simulink model "system_20220515_1_sm_master"  (R2020b)
settings: Solver=ode4  StartTime=0.0  StopTime=inf  FixedStep=0.001  RelTol=1e-3  EnableMultiTasking=on
PreLoadFcn:
  | simulation_vars
PostLoadFcn:
  | simulation_vars
InitFcn:
  | simulation_vars
StartFcn:
  | simulation_vars
undefined symbols (not defined in the file or in its folder): ang_variance, bus_va_seed, bus_vm_seed, en_spoofing_attack, event_time_end, event_time_start, line_iang0_seed, line_iang1_seed, line_imag0_seed, line_imag1_seed, mag_variance, spoof_lower_limit, spoof_upper_limit, Ts, xf_iang0_seed, xf_iang1_seed, xf_imag0_seed, xf_imag1_seed
libraries: rtlab x209, simulink x21, opal_lib x3, rtlab_phasor x1, rtio_spectracom x1
(part 4 of 4)

== system system_20220515_1_sm_master/sm_master/PMU207_signals/Spoofing attack ==
  note: Modify demux and mux to fit input size.
      | Only modifies the angle measurements.
  Input : Inport
  Add : Sum
  Constant : Constant  Value=en_spoofing_attack.pmu_207
  Demux : Demux
  Demux1 : Demux  Outputs=2
  Multiply : Product
  Mux : Mux
  Mux1 : Mux  Inputs=2
  Ramp : simulink/Sources/Ramp  slope=1*pi()/180  start=spoof_st.pmu_207  InitialOutput=0
  Saturation : Saturate  UpperLimit=spoof_upper_limit  LowerLimit=spoof_lower_limit
  Output : Outport  VectorParamsAs1DForOutWhenUnconnected=off
  wires:
  Multiply/1 -> Add/1
  Saturation/1 -> Multiply/1
  Constant/1 -> Multiply/2
  Ramp/1 -> Saturation/1
  Input/1 -> Demux/1
  Mux/1 -> Output/1
  Demux/1 -> Mux/1
  Demux/3 -> Mux/3
  Demux/4 -> Mux1/2
  Demux/2 -> Mux1/1
  Mux1/1 -> Add/2
  Add/1 -> Demux1/1
  Demux1/1 -> Mux/2
  Demux1/2 -> Mux/4

== system system_20220515_1_sm_master/sm_master/PMU210_signals/Spoofing attack ==
  note: Modify demux and mux to fit input size.
      | Only modifies the angle measurements.
  Input : Inport
  Add : Sum
  Constant : Constant  Value=en_spoofing_attack.pmu_210
  Demux : Demux  Outputs=12
  Demux1 : Demux  Outputs=6
  Multiply : Product
  Mux : Mux  Inputs=12
  Mux1 : Mux  Inputs=6
  Ramp : simulink/Sources/Ramp  slope=1*pi()/180  start=spoof_st.pmu_210  InitialOutput=0
  Saturation : Saturate  UpperLimit=spoof_upper_limit  LowerLimit=spoof_lower_limit
  Output : Outport  VectorParamsAs1DForOutWhenUnconnected=off
  wires:
  Multiply/1 -> Add/1
  Saturation/1 -> Multiply/1
  Constant/1 -> Multiply/2
  Ramp/1 -> Saturation/1
  Input/1 -> Demux/1
  Mux/1 -> Output/1
  Demux/1 -> Mux/1
  Demux/3 -> Mux/3
  Demux/5 -> Mux/5
  Demux/7 -> Mux/7
  Demux/9 -> Mux/9
  Demux/10 -> Mux1/5
  Demux/8 -> Mux1/4
  Demux/6 -> Mux1/3
  Demux/4 -> Mux1/2
  Demux/2 -> Mux1/1
  Mux1/1 -> Add/2
  Add/1 -> Demux1/1
  Demux1/1 -> Mux/2
  Demux1/2 -> Mux/4
  Demux1/3 -> Mux/6
  Demux1/4 -> Mux/8
  Demux1/5 -> Mux/10
  Demux/11 -> Mux/11
  Demux/12 -> Mux1/6
  Demux1/6 -> Mux/12

== system system_20220515_1_sm_master/sm_master/PMU216_signals/Spoofing attack ==
  note: Modify demux and mux to fit input size.
      | Only modifies the angle measurements.
  Input : Inport
  Add : Sum
  Constant : Constant  Value=en_spoofing_attack.pmu_216
  Demux : Demux  Outputs=10
  Demux1 : Demux  Outputs=5
  Multiply : Product
  Mux : Mux  Inputs=10
  Mux1 : Mux  Inputs=5
  Ramp : simulink/Sources/Ramp  slope=1*pi()/180  start=spoof_st.pmu_216  InitialOutput=0
  Saturation : Saturate  UpperLimit=spoof_upper_limit  LowerLimit=spoof_lower_limit
  Output : Outport  VectorParamsAs1DForOutWhenUnconnected=off
  wires:
  Multiply/1 -> Add/1
  Saturation/1 -> Multiply/1
  Constant/1 -> Multiply/2
  Ramp/1 -> Saturation/1
  Input/1 -> Demux/1
  Mux/1 -> Output/1
  Demux/1 -> Mux/1
  Demux/3 -> Mux/3
  Demux/5 -> Mux/5
  Demux/7 -> Mux/7
  Demux/9 -> Mux/9
  Demux/10 -> Mux1/5
  Demux/8 -> Mux1/4
  Demux/6 -> Mux1/3
  Demux/4 -> Mux1/2
  Demux/2 -> Mux1/1
  Mux1/1 -> Add/2
  Add/1 -> Demux1/1
  Demux1/1 -> Mux/2
  Demux1/2 -> Mux/4
  Demux1/3 -> Mux/6
  Demux1/4 -> Mux/8
  Demux1/5 -> Mux/10

== system system_20220515_1_sm_master/sm_master/PMU221_signals/Spoofing attack ==
  note: Modify demux and mux to fit input size.
      | Only modifies the angle measurements.
  Input : Inport
  Add : Sum
  Constant : Constant  Value=en_spoofing_attack.pmu_221
  Demux : Demux  Outputs=12
  Demux1 : Demux  Outputs=6
  Multiply : Product
  Mux : Mux  Inputs=12
  Mux1 : Mux  Inputs=6
  Ramp : simulink/Sources/Ramp  slope=1*pi()/180  start=spoof_st.pmu_221  InitialOutput=0
  Saturation : Saturate  UpperLimit=spoof_upper_limit  LowerLimit=spoof_lower_limit
  Output : Outport  VectorParamsAs1DForOutWhenUnconnected=off
  wires:
  Multiply/1 -> Add/1
  Saturation/1 -> Multiply/1
  Constant/1 -> Multiply/2
  Ramp/1 -> Saturation/1
  Input/1 -> Demux/1
  Mux/1 -> Output/1
  Demux/1 -> Mux/1
  Demux/3 -> Mux/3
  Demux/5 -> Mux/5
  Demux/7 -> Mux/7
  Demux/9 -> Mux/9
  Demux/10 -> Mux1/5
  Demux/8 -> Mux1/4
  Demux/6 -> Mux1/3
  Demux/4 -> Mux1/2
  Demux/2 -> Mux1/1
  Mux1/1 -> Add/2
  Add/1 -> Demux1/1
  Demux1/1 -> Mux/2
  Demux1/2 -> Mux/4
  Demux1/3 -> Mux/6
  Demux1/4 -> Mux/8
  Demux1/5 -> Mux/10
  Demux/11 -> Mux/11
  Demux/12 -> Mux1/6
  Demux1/6 -> Mux/12

== system system_20220515_1_sm_master/sm_master/PMU223_signals/Spoofing attack ==
  note: Modify demux and mux to fit input size.
      | Only modifies the angle measurements.
  Input : Inport
  Add : Sum
  Constant : Constant  Value=en_spoofing_attack.pmu_223
  Demux : Demux  Outputs=12
  Demux1 : Demux  Outputs=6
  Multiply : Product
  Mux : Mux  Inputs=12
  Mux1 : Mux  Inputs=6
  Ramp : simulink/Sources/Ramp  slope=1*pi()/180  start=spoof_st.pmu_223  InitialOutput=0
  Saturation : Saturate  UpperLimit=spoof_upper_limit  LowerLimit=spoof_lower_limit
  Output : Outport  VectorParamsAs1DForOutWhenUnconnected=off
  wires:
  Multiply/1 -> Add/1
  Saturation/1 -> Multiply/1
  Constant/1 -> Multiply/2
  Ramp/1 -> Saturation/1
  Input/1 -> Demux/1
  Mux/1 -> Output/1
  Demux/1 -> Mux/1
  Demux/3 -> Mux/3
  Demux/5 -> Mux/5
  Demux/7 -> Mux/7
  Demux/9 -> Mux/9
  Demux/10 -> Mux1/5
  Demux/8 -> Mux1/4
  Demux/6 -> Mux1/3
  Demux/4 -> Mux1/2
  Demux/2 -> Mux1/1
  Mux1/1 -> Add/2
  Add/1 -> Demux1/1
  Demux1/1 -> Mux/2
  Demux1/2 -> Mux/4
  Demux1/3 -> Mux/6
  Demux1/4 -> Mux/8
  Demux1/5 -> Mux/10
  Demux/11 -> Mux/11
  Demux/12 -> Mux1/6
  Demux1/6 -> Mux/12

== system system_20220515_1_sm_master/sm_master/PMU302_signals/Spoofing attack ==
  note: Modify demux and mux to fit input size.
      | Only modifies the angle measurements.
  Input : Inport
  Add : Sum
  Constant : Constant  Value=en_spoofing_attack.pmu_302
  Demux : Demux  Outputs=8
  Demux1 : Demux
  Multiply : Product
  Mux : Mux  Inputs=8
  Mux1 : Mux
  Ramp : simulink/Sources/Ramp  slope=1*pi()/180  start=spoof_st.pmu_302  InitialOutput=0
  Saturation : Saturate  UpperLimit=spoof_upper_limit  LowerLimit=spoof_lower_limit
  Output : Outport  VectorParamsAs1DForOutWhenUnconnected=off
  wires:
  Multiply/1 -> Add/1
  Saturation/1 -> Multiply/1
  Constant/1 -> Multiply/2
  Ramp/1 -> Saturation/1
  Input/1 -> Demux/1
  Mux/1 -> Output/1
  Demux/1 -> Mux/1
  Demux/3 -> Mux/3
  Demux/5 -> Mux/5
  Demux/7 -> Mux/7
  Demux/8 -> Mux1/4
  Demux/6 -> Mux1/3
  Demux/4 -> Mux1/2
  Demux/2 -> Mux1/1
  Mux1/1 -> Add/2
  Add/1 -> Demux1/1
  Demux1/1 -> Mux/2
  Demux1/2 -> Mux/4
  Demux1/3 -> Mux/6
  Demux1/4 -> Mux/8

== system system_20220515_1_sm_master/sm_master/PMU303_signals/Spoofing attack ==
  note: Modify demux and mux to fit input size.
      | Only modifies the angle measurements.
  Input : Inport
  Add : Sum
  Constant : Constant  Value=en_spoofing_attack.pmu_303
  Demux : Demux  Outputs=8
  Demux1 : Demux
  Multiply : Product
  Mux : Mux  Inputs=8
  Mux1 : Mux
  Ramp : simulink/Sources/Ramp  slope=1*pi()/180  start=spoof_st.pmu_303  InitialOutput=0
  Saturation : Saturate  UpperLimit=spoof_upper_limit  LowerLimit=spoof_lower_limit
  Output : Outport  VectorParamsAs1DForOutWhenUnconnected=off
  wires:
  Multiply/1 -> Add/1
  Saturation/1 -> Multiply/1
  Constant/1 -> Multiply/2
  Ramp/1 -> Saturation/1
  Input/1 -> Demux/1
  Mux/1 -> Output/1
  Demux/1 -> Mux/1
  Demux/3 -> Mux/3
  Demux/5 -> Mux/5
  Demux/7 -> Mux/7
  Demux/8 -> Mux1/4
  Demux/6 -> Mux1/3
  Demux/4 -> Mux1/2
  Demux/2 -> Mux1/1
  Mux1/1 -> Add/2
  Add/1 -> Demux1/1
  Demux1/1 -> Mux/2
  Demux1/2 -> Mux/4
  Demux1/3 -> Mux/6
  Demux1/4 -> Mux/8

== system system_20220515_1_sm_master/sm_master/PMU307_signals/Spoofing attack ==
  note: Modify demux and mux to fit input size.
      | Only modifies the angle measurements.
  Input : Inport
  Add : Sum
  Constant : Constant  Value=en_spoofing_attack.pmu_307
  Demux : Demux
  Demux1 : Demux  Outputs=2
  Multiply : Product
  Mux : Mux
  Mux1 : Mux  Inputs=2
  Ramp : simulink/Sources/Ramp  slope=1*pi()/180  start=spoof_st.pmu_307  InitialOutput=0
  Saturation : Saturate  UpperLimit=spoof_upper_limit  LowerLimit=spoof_lower_limit
  Output : Outport  VectorParamsAs1DForOutWhenUnconnected=off
  wires:
  Multiply/1 -> Add/1
  Saturation/1 -> Multiply/1
  Constant/1 -> Multiply/2
  Ramp/1 -> Saturation/1
  Input/1 -> Demux/1
  Mux/1 -> Output/1
  Demux/1 -> Mux/1
  Demux/3 -> Mux/3
  Demux/4 -> Mux1/2
  Demux/2 -> Mux1/1
  Mux1/1 -> Add/2
  Add/1 -> Demux1/1
  Demux1/1 -> Mux/2
  Demux1/2 -> Mux/4

== system system_20220515_1_sm_master/sm_master/PMU310_signals/Spoofing attack ==
  note: Modify demux and mux to fit input size.
      | Only modifies the angle measurements.
  Input : Inport
  Add : Sum
  Constant : Constant  Value=en_spoofing_attack.pmu_310
  Demux : Demux  Outputs=12
  Demux1 : Demux  Outputs=6
  Multiply : Product
  Mux : Mux  Inputs=12
  Mux1 : Mux  Inputs=6
  Ramp : simulink/Sources/Ramp  slope=1*pi()/180  start=spoof_st.pmu_310  InitialOutput=0
  Saturation : Saturate  UpperLimit=spoof_upper_limit  LowerLimit=spoof_lower_limit
  Output : Outport  VectorParamsAs1DForOutWhenUnconnected=off
  wires:
  Multiply/1 -> Add/1
  Saturation/1 -> Multiply/1
  Constant/1 -> Multiply/2
  Ramp/1 -> Saturation/1
  Input/1 -> Demux/1
  Mux/1 -> Output/1
  Demux/1 -> Mux/1
  Demux/3 -> Mux/3
  Demux/5 -> Mux/5
  Demux/7 -> Mux/7
  Demux/9 -> Mux/9
  Demux/10 -> Mux1/5
  Demux/8 -> Mux1/4
  Demux/6 -> Mux1/3
  Demux/4 -> Mux1/2
  Demux/2 -> Mux1/1
  Mux1/1 -> Add/2
  Add/1 -> Demux1/1
  Demux1/1 -> Mux/2
  Demux1/2 -> Mux/4
  Demux1/3 -> Mux/6
  Demux1/4 -> Mux/8
  Demux1/5 -> Mux/10
  Demux/11 -> Mux/11
  Demux/12 -> Mux1/6
  Demux1/6 -> Mux/12

== system system_20220515_1_sm_master/sm_master/PMU316_signals/Spoofing attack ==
  note: Modify demux and mux to fit input size.
      | Only modifies the angle measurements.
  Input : Inport
  Add : Sum
  Constant : Constant  Value=en_spoofing_attack.pmu_316
  Demux : Demux  Outputs=10
  Demux1 : Demux  Outputs=5
  Multiply : Product
  Mux : Mux  Inputs=10
  Mux1 : Mux  Inputs=5
  Ramp : simulink/Sources/Ramp  slope=1*pi()/180  start=spoof_st.pmu_316  InitialOutput=0
  Saturation : Saturate  UpperLimit=spoof_upper_limit  LowerLimit=spoof_lower_limit
  Output : Outport  VectorParamsAs1DForOutWhenUnconnected=off
  wires:
  Multiply/1 -> Add/1
  Saturation/1 -> Multiply/1
  Constant/1 -> Multiply/2
  Ramp/1 -> Saturation/1
  Input/1 -> Demux/1
  Mux/1 -> Output/1
  Demux/1 -> Mux/1
  Demux/3 -> Mux/3
  Demux/5 -> Mux/5
  Demux/7 -> Mux/7
  Demux/9 -> Mux/9
  Demux/10 -> Mux1/5
  Demux/8 -> Mux1/4
  Demux/6 -> Mux1/3
  Demux/4 -> Mux1/2
  Demux/2 -> Mux1/1
  Mux1/1 -> Add/2
  Add/1 -> Demux1/1
  Demux1/1 -> Mux/2
  Demux1/2 -> Mux/4
  Demux1/3 -> Mux/6
  Demux1/4 -> Mux/8
  Demux1/5 -> Mux/10

== system system_20220515_1_sm_master/sm_master/PMU321_signals/Spoofing attack ==
  note: Modify demux and mux to fit input size.
      | Only modify the angle measurements.
  Input : Inport
  Add : Sum
  Constant : Constant  Value=en_spoofing_attack.pmu_321
  Demux : Demux  Outputs=12
  Demux1 : Demux  Outputs=6
  Multiply : Product
  Mux : Mux  Inputs=12
  Mux1 : Mux  Inputs=6
  Ramp : simulink/Sources/Ramp  slope=1*pi()/180  start=spoof_st.pmu_321  InitialOutput=0
  Saturation : Saturate  UpperLimit=spoof_upper_limit  LowerLimit=spoof_lower_limit
  Output : Outport  VectorParamsAs1DForOutWhenUnconnected=off
  wires:
  Multiply/1 -> Add/1
  Saturation/1 -> Multiply/1
  Constant/1 -> Multiply/2
  Ramp/1 -> Saturation/1
  Input/1 -> Demux/1
  Mux/1 -> Output/1
  Demux/1 -> Mux/1
  Demux/3 -> Mux/3
  Demux/5 -> Mux/5
  Demux/7 -> Mux/7
  Demux/9 -> Mux/9
  Demux/11 -> Mux/11
  Demux/12 -> Mux1/6
  Demux/10 -> Mux1/5
  Demux/8 -> Mux1/4
  Demux/6 -> Mux1/3
  Demux/4 -> Mux1/2
  Demux/2 -> Mux1/1
  Mux1/1 -> Add/2
  Add/1 -> Demux1/1
  Demux1/1 -> Mux/2
  Demux1/2 -> Mux/4
  Demux1/3 -> Mux/6
  Demux1/4 -> Mux/8
  Demux1/5 -> Mux/10
  Demux1/6 -> Mux/12

== system system_20220515_1_sm_master/sm_master/PMU323_signals/Spoofing attack ==
  note: Modify demux and mux to fit input size.
      | Only modify the angle measurements.
  Input : Inport
  Add : Sum
  Constant : Constant  Value=en_spoofing_attack.pmu_323
  Demux : Demux  Outputs=12
  Demux1 : Demux  Outputs=6
  Multiply : Product
  Mux : Mux  Inputs=12
  Mux1 : Mux  Inputs=6
  Ramp : simulink/Sources/Ramp  slope=1*pi()/180  start=spoof_st.pmu_323  InitialOutput=0
  Saturation : Saturate  UpperLimit=spoof_upper_limit  LowerLimit=spoof_lower_limit
  Output : Outport  VectorParamsAs1DForOutWhenUnconnected=off
  wires:
  Multiply/1 -> Add/1
  Saturation/1 -> Multiply/1
  Constant/1 -> Multiply/2
  Ramp/1 -> Saturation/1
  Input/1 -> Demux/1
  Mux/1 -> Output/1
  Demux/1 -> Mux/1
  Demux/3 -> Mux/3
  Demux/5 -> Mux/5
  Demux/7 -> Mux/7
  Demux/9 -> Mux/9
  Demux/11 -> Mux/11
  Demux/12 -> Mux1/6
  Demux/10 -> Mux1/5
  Demux/8 -> Mux1/4
  Demux/6 -> Mux1/3
  Demux/4 -> Mux1/2
  Demux/2 -> Mux1/1
  Mux1/1 -> Add/2
  Add/1 -> Demux1/1
  Demux1/1 -> Mux/2
  Demux1/2 -> Mux/4
  Demux1/3 -> Mux/6
  Demux1/4 -> Mux/8
  Demux1/5 -> Mux/10
  Demux1/6 -> Mux/12

== system system_20220515_1_sm_master/sm_master/rtlab_send_subsystem/Subsystem1 ==
  In1 : Inport
  In2 : Inport  Port=2
  In3 : Inport  Port=3
  In4 : Inport  Port=4
  Mux : Mux
  Send1 : opal_lib/Communication/OpSendToNT  Acqu_group=1
  wires:
  Mux/1 -> Send1/1
  In1/1 -> Mux/1
  In2/1 -> Mux/2
  In3/1 -> Mux/3
  In4/1 -> Mux/4

== matlab function system_20220515_1_sm_master/sm_master/bus_va_noise/MATLAB Function ==
  data: u input; y output
function y = wrap_angle(u)

max_val = 180;
min_val = -179.99;

if u > max_val
    u = u - round(u/(2*max_val))*max_val*2;
end

if u < min_val
    u = u + round(abs(u)/(2*max_val))*max_val*2;
end

y = u;

== matlab function system_20220515_1_sm_master/sm_master/line_iang1_noise/MATLAB Function ==
  data: u input; y output
function y = wrap_angle(u)

max_val = 180;
min_val = -179.99;

if u > max_val
    u = u - round(u/(2*max_val))*max_val*2;
end

if u < min_val
    u = u + round(abs(u)/(2*max_val))*max_val*2;
end

y = u;

== matlab function system_20220515_1_sm_master/sm_master/xf_iang0_noise/MATLAB Function ==
  data: u input; y output
function y = wrap_angle(u)

max_val = 180;
min_val = -179.99;

if u > max_val
    u = u - round(u/(2*max_val))*max_val*2;
end

if u < min_val
    u = u + round(abs(u)/(2*max_val))*max_val*2;
end

y = u;

== matlab function system_20220515_1_sm_master/sm_master/xf_iang1_noise/MATLAB Function ==
  data: u input; y output
function y = wrap_angle(u)

max_val = 180;
min_val = -179.99;

if u > max_val
    u = u - round(u/(2*max_val))*max_val*2;
end

if u < min_val
    u = u + round(abs(u)/(2*max_val))*max_val*2;
end

y = u;

== matlab function system_20220515_1_sm_master/sm_master/line_iang0_noise/MATLAB Function ==
  data: u input; y output
function y = wrap_angle(u)

max_val = 180;
min_val = -179.99;

if u > max_val
    u = u - round(u/(2*max_val))*max_val*2;
end

if u < min_val
    u = u + round(abs(u)/(2*max_val))*max_val*2;
end

y = u;
